simulink model "BallOnBeam_Model_Controller"  (R2018b)
settings: Solver=VariableStepAuto  StartTime=0.0  StopTime=5*ts  MaxStep=1e-3  MinStep=1e-4  RelTol=1e-3
values from neighbouring files (symbols this model uses):
  A = [0 0 1 0 ... (first row only)    [Main.m]
  B = [0;0;K1;0]    [Main.m]
  C = [0, 1, 0, 0]    [Main.m]
  D = 0    [Main.m]
  Kc = real(place(A,B,[p1,p2,-20,-40]))    [Main.m]
  x10 = 0    [Main.m]
  x20 = 0    [Main.m]
  x30 = 0    [Main.m]
  x40 = 0    [Main.m]
libraries: vrlib x3
settings Model: Creator=Eduardo  LastModifiedBy=ohara
settings SolverCC: InitialStep=1e-3

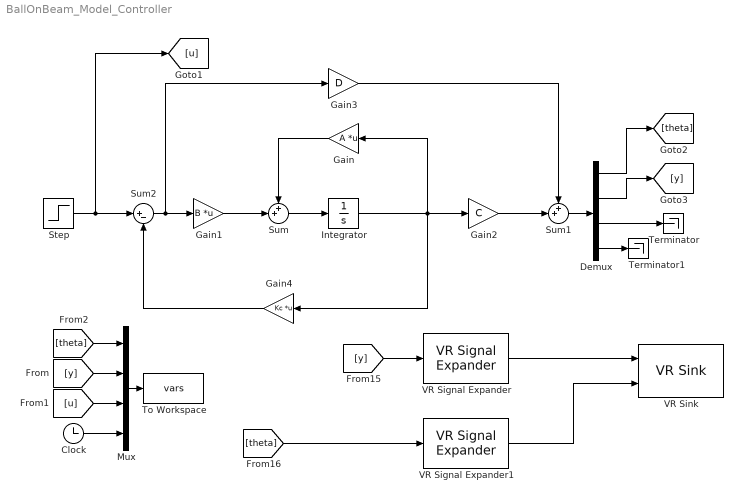
== system BallOnBeam_Model_Controller ==
  Clock : Clock
  Demux : Demux
  Gain : Gain  Gain=A  Multiplication=Matrix(K*u)
  Gain1 : Gain  Gain=B  Multiplication=Matrix(K*u)
  Gain2 : Gain  Gain=C
  Gain3 : Gain  Gain=D
  Gain4 : Gain  Gain=Kc  Multiplication=Matrix(K*u)
  Integrator : Integrator  InitialCondition=[x10;x20;x30;x40]
  Mux : Mux
  Step : Step  SampleTime=0
  Sum : Sum  Inputs=++|
  Sum1 : Sum  Inputs=++|
  Sum2 : Sum  Inputs=|+-
  Terminator : Terminator
  Terminator1 : Terminator
  To Workspace : ToWorkspace  VariableName=vars  SaveFormat=Timeseries  SampleTime=-1
  VR Signal Expander : vrlib/VR Signal Expander  outwidth=3  outidx=[1]
      settings: SourceProductName=Simulink 3D Animation  SourceProductBaseCode=VR
  VR Signal Expander1 : vrlib/VR Signal Expander  outwidth=4  outidx=[4 3]
      settings: SourceProductName=Simulink 3D Animation  SourceProductBaseCode=VR
  VR Sink : vrlib/VR Sink  InstantiateOnLoad=on  SampleTime=0.01  ViewEnable=on  RemoteChange=off  RemoteView=off  FieldsWritten=Ball.translation.3.1.1.double#Rod.rotation.4.1.1.double  WorldFileName=ballonbeam_3danim.WRL  AutoView=off  VideoDimensions=[]  AllowVariableSize=off
      settings: SourceProductBaseCode=VR
  wires:
  Gain1/1 -> Sum/2
  Sum/1 -> Integrator/1
  Gain/1 -> Sum/1
  Integrator/1 -> Gain4/1, Gain2/1, Gain/1
  Gain2/1 -> Sum1/2
  Gain3/1 -> Sum1/1
  Sum2/1 -> Gain3/1, Gain1/1
  Step/1 -> [u], Sum2/1
  Gain4/1 -> Sum2/2
  Mux/1 -> To Workspace/1
  [theta] -> VR Signal Expander1/1
  VR Signal Expander1/1 -> VR Sink/2
  VR Signal Expander/1 -> VR Sink/1
  [y] -> VR Signal Expander/1
  Demux/1 -> [theta]
  Sum1/1 -> Demux/1
  Demux/2 -> [y]
  Demux/3 -> Terminator/1
  Demux/4 -> Terminator1/1
  Clock/1 -> Mux/4
  [u] -> Mux/3
  [y] -> Mux/2
  [theta] -> Mux/1
